simulink model "slc_ut"  (Simulink 8.1)
settings: Solver=FixedStepDiscrete  StartTime=0.0  StopTime=10  FixedStep=0.005  RelTol=1e-3
PostLoadFcn:
  | , if any(exist('dsrtsu_mdlpostloadfcn', 'file') == [2, 3, 6]), try dsrtsu_mdlpostloadfcn('Execute', bdroot); catch fprintf('Error in PostLoadFcn (dsrtsu_mdlpostloadfcn) for model "%s":\n %s\n', bdroot, lasterr); end, end,
libraries: siltestlib x20, slc x1
settings Model: DSRTSU_INTERNAL_RTI_VER=450  DSRTSU_INTERNAL_RTI_TYPE=rti1401  RTICANMMDATA=struct('GeneralSetupData',struct('modelroot','D:\ELN150201_TAIWAN\trunk\AdasDragon\software\sw_development\arch\app\acc','generalsettings',struct('filesettings',struct('destfolder',struct('Name','RTICANMM_FILES','Check',1),'buildfolder',struct('Name','.','Check',1),'AbsDestfolder',struct('Name','D:\ELN150201_TAIWAN\trunk\AdasDragon\software\sw_development\arch\app\acc\RTICANMM_FILES'),'AbsBuildfolder',struct('Name','D:\ELN150201_TAIWAN\trunk\AdasDragon\software\sw_development\arch\app\acc'))),'options',struct('addpaths',1,'rmpaths',1,'addtrcexclusion',logical(1),'cannavigator',struct('checkmonitoring',0),'show_usrtrc',0,'use_usrtrc',0),'advanced',struct('options',[1 1 1 1 1 1 1 1 1 1 1 1 1 1 1 1 1 1 1 1 1 1 1 1 1 1 1 1 1 1 1 1 1 1 1 1 1 1 1 1 1 1 1 1 1 1 1 1 1 1 1 1 1 1 1 1 1 1 1 1 1 1 1 1 1 1 1 1 1 1 1 1 1 1 1 1 1 1 1 1 1 1 1 1 1 1 1 1 1 1 1 1 1 1 1 1 1 1 1 1]),'MPSetup',{{}},'modelname','slc_ut','block','slc_ut'))  DSRTSU_INTERNAL_RTIFPGA=40  Creator=AT015411  LastModifiedBy=AT015555  BufferReuse=off
settings DataIOCC: SignalLoggingSaveFormat=Dataset
settings OptimizationCC: BlockReduction=off  OptimizeBlockIOStorage=off  BufferReuse=off  ExpressionFolding=off  ExpressionDepthLimit=128  LocalBlockOutputs=off
settings DebuggingCC: FcnCallInpInsideContextMsg=EnableAllAsError
settings HardwareCC: ProdIntDivRoundTo=Zero  ProdEndianess=BigEndian  ProdHWDeviceType=Generic->Custom  TargetIntDivRoundTo=Zero  TargetEndianess=BigEndian  TargetHWDeviceType=Generic->Custom
settings RTWCC: SystemTargetFile=rti1005.tlc  MakeCommand=make_rti  TemplateMakefile=rti1005.tmf  Description=dSPACE DS1005 Hardware Platform  ProcessScript=rti1005_make_rtw_hook
settings STFCustomTargetCC: CodeReplacementLibrary=ANSI_C  ParMdlRefBuildCompliant=on  GeneratePreprocessorConditionals=Disable all  MatFileLogging=on  SystemTargetFile=rti1005.tlc
settings GRTTargetCC: CompOptLevelCompliant=off  ConcurrentExecutionCompliant=off  ExtModeMexFile=noextcomm
settings CustomProperty: DataType=RTWOptions_EnumType_C__Program Files (x86)_dSPACE RCPHIL 2014-B_MATLAB_RTI_RTI1401_TLC_rti1005_1InitialSimState  Value=RUN
settings EnumStrPairs: String=RUN

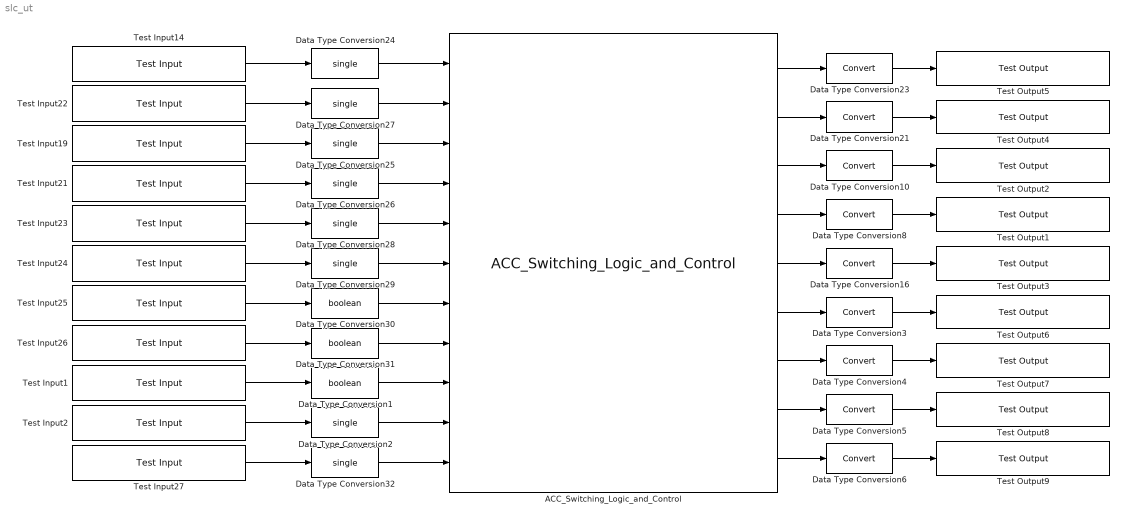
== system slc_ut ==
  ACC_Switching_Logic_and_Control : slc/ACC_Switching_Logic_and_Control
  Data Type Conversion1 : DataTypeConversion  OutDataTypeStr=boolean
  Data Type Conversion{3..6,8,10,16,21,23} (9 alike) : DataTypeConversion
  Data Type Conversion{2,24..29,32} (8 alike) : DataTypeConversion  OutDataTypeStr=single
  Data Type Conversion30 : DataTypeConversion  OutDataTypeStr=boolean
  Data Type Conversion31 : DataTypeConversion  OutDataTypeStr=boolean
  Test Input1 : siltestlib/Test Input  varname=VACC_ACCOverride_flg  sampletime=0.005
  Test Input14 : siltestlib/Test Input  varname=VACC_VehSpd_mps  sampletime=0.005
  Test Input19 : siltestlib/Test Input  varname=VJUD_ACCSetTimeGap_s  sampletime=0.005
  Test Input2 : siltestlib/Test Input  varname=VIFO_ACCMCLongAcc_mps2  sampletime=0.005
  Test Input21 : siltestlib/Test Input  varname=VIFO_ACCTargetVehRelSpeedX_mps  sampletime=0.005
  Test Input22 : siltestlib/Test Input  varname=VJUD_ACCSetSpeed_kph  sampletime=0.005
  Test Input23 : siltestlib/Test Input  varname=VACC_ACCTargetVehSpd_mps  sampletime=0.005
  Test Input24 : siltestlib/Test Input  varname=VIFO_ACCTGap_s  sampletime=0.005
  Test Input25 : siltestlib/Test Input  varname=VACC_ACCTargetVehAssigned_flg  sampletime=0.005
  Test Input26 : siltestlib/Test Input  varname=VIFO_ACCDist_flg  sampletime=0.005
  Test Input27 : siltestlib/Test Input  varname=VIFO_ACCVehClearance_m  sampletime=0.005
  Test Output1 : siltestlib/Test Output  varname=VACC_DesiredDistance_m  sampletime=-1
  Test Output2 : siltestlib/Test Output  varname=VACC_DecelControlReq_flg  sampletime=-1
  Test Output3 : siltestlib/Test Output  varname=VACC_ACCDistControlSel_flg  sampletime=-1
  Test Output4 : siltestlib/Test Output  varname=VACC_ACCRefSpd_mps  sampletime=-1
  Test Output5 : siltestlib/Test Output  varname=VACC_TorqueReleaseReq_flg  sampletime=-1
  Test Output6 : siltestlib/Test Output  varname=VACC_ACCBrakeToStop_flg  sampletime=-1
  Test Output7 : siltestlib/Test Output  varname=VACC_ACCMCBraking_flg  sampletime=-1
  Test Output8 : siltestlib/Test Output  varname=VACC_ACCMCDecel_mps2  sampletime=-1
  Test Output9 : siltestlib/Test Output  varname=VACC_ACCBrakeReleaseSituation_flg  sampletime=-1
  wires:
  Data Type Conversion8/1 -> Test Output1/1
  Data Type Conversion10/1 -> Test Output2/1
  Data Type Conversion16/1 -> Test Output3/1
  Data Type Conversion21/1 -> Test Output4/1
  Data Type Conversion23/1 -> Test Output5/1
  Test Input14/1 -> Data Type Conversion24/1
  Data Type Conversion24/1 -> ACC_Switching_Logic_and_Control/1
  Test Input19/1 -> Data Type Conversion25/1
  Data Type Conversion25/1 -> ACC_Switching_Logic_and_Control/3
  Test Input21/1 -> Data Type Conversion26/1
  Data Type Conversion26/1 -> ACC_Switching_Logic_and_Control/4
  Test Input22/1 -> Data Type Conversion27/1
  Data Type Conversion27/1 -> ACC_Switching_Logic_and_Control/2
  Test Input23/1 -> Data Type Conversion28/1
  Data Type Conversion28/1 -> ACC_Switching_Logic_and_Control/5
  Test Input24/1 -> Data Type Conversion29/1
  Data Type Conversion29/1 -> ACC_Switching_Logic_and_Control/6
  Test Input25/1 -> Data Type Conversion30/1
  Data Type Conversion30/1 -> ACC_Switching_Logic_and_Control/7
  Test Input26/1 -> Data Type Conversion31/1
  Data Type Conversion31/1 -> ACC_Switching_Logic_and_Control/8
  Test Input27/1 -> Data Type Conversion32/1
  Test Input1/1 -> Data Type Conversion1/1
  Data Type Conversion1/1 -> ACC_Switching_Logic_and_Control/9
  Test Input2/1 -> Data Type Conversion2/1
  Data Type Conversion2/1 -> ACC_Switching_Logic_and_Control/10
  Data Type Conversion32/1 -> ACC_Switching_Logic_and_Control/11
  Data Type Conversion3/1 -> Test Output6/1
  Data Type Conversion4/1 -> Test Output7/1
  Data Type Conversion5/1 -> Test Output8/1
  Data Type Conversion6/1 -> Test Output9/1
  ACC_Switching_Logic_and_Control/1 -> Data Type Conversion23/1
  ACC_Switching_Logic_and_Control/2 -> Data Type Conversion21/1
  ACC_Switching_Logic_and_Control/3 -> Data Type Conversion10/1
  ACC_Switching_Logic_and_Control/4 -> Data Type Conversion8/1
  ACC_Switching_Logic_and_Control/5 -> Data Type Conversion16/1
  ACC_Switching_Logic_and_Control/6 -> Data Type Conversion3/1
  ACC_Switching_Logic_and_Control/7 -> Data Type Conversion4/1
  ACC_Switching_Logic_and_Control/8 -> Data Type Conversion5/1
  ACC_Switching_Logic_and_Control/9 -> Data Type Conversion6/1
